simulink library "pixhawk_slib_swarm"  (R2022b)
settings: Solver=ode45  StartTime=0.0  StopTime=10.0  RelTol=1e-3
libraries: $bdroot x3, etargetslib x2, simulink x2
(part 2 of 2)

== system pixhawk_slib_swarm/RealCtrl28D/getMask6 ==
  In1 : Inport
  In2 : Inport  Port=2
  Data Type Conversion6 : DataTypeConversion  OutDataTypeStr=uint32  SaturateOnIntegerOverflow=off  RndMeth=Floor
  IgnoreAll : Constant  Value=bin2dec('1111111111111111')
  Switch : Switch  Criteria=u2 > Threshold  SaturateOnIntegerOverflow=off  InputSameDT=off
  Out1 : Outport  VectorParamsAs1DForOutWhenUnconnected=off
  wires:
  In1/1 -> Switch/2
  Switch/1 -> Data Type Conversion6/1
  Data Type Conversion6/1 -> Out1/1
  IgnoreAll/1 -> Switch/3
  In2/1 -> Switch/1

== system pixhawk_slib_swarm/RealCtrl28D/getMask7 ==
  In1 : Inport
  In2 : Inport  Port=2
  Data Type Conversion6 : DataTypeConversion  OutDataTypeStr=uint32  SaturateOnIntegerOverflow=off  RndMeth=Floor
  IgnoreAll : Constant  Value=bin2dec('1111111111111111')
  Switch : Switch  Criteria=u2 > Threshold  SaturateOnIntegerOverflow=off  InputSameDT=off
  Out1 : Outport  VectorParamsAs1DForOutWhenUnconnected=off
  wires:
  In1/1 -> Switch/2
  Switch/1 -> Data Type Conversion6/1
  Data Type Conversion6/1 -> Out1/1
  IgnoreAll/1 -> Switch/3
  In2/1 -> Switch/1

== system pixhawk_slib_swarm/RealCtrl28D/getMask8 ==
  In1 : Inport
  In2 : Inport  Port=2
  Data Type Conversion6 : DataTypeConversion  OutDataTypeStr=uint32  SaturateOnIntegerOverflow=off  RndMeth=Floor
  IgnoreAll : Constant  Value=bin2dec('1111111111111111')
  Switch : Switch  Criteria=u2 > Threshold  SaturateOnIntegerOverflow=off  InputSameDT=off
  Out1 : Outport  VectorParamsAs1DForOutWhenUnconnected=off
  wires:
  In1/1 -> Switch/2
  Switch/1 -> Data Type Conversion6/1
  Data Type Conversion6/1 -> Out1/1
  IgnoreAll/1 -> Switch/3
  In2/1 -> Switch/1

== system pixhawk_slib_swarm/RealCtrl28D/getMask9 ==
  In1 : Inport
  In2 : Inport  Port=2
  Data Type Conversion6 : DataTypeConversion  OutDataTypeStr=uint32  SaturateOnIntegerOverflow=off  RndMeth=Floor
  IgnoreAll : Constant  Value=bin2dec('1111111111111111')
  Switch : Switch  Criteria=u2 > Threshold  SaturateOnIntegerOverflow=off  InputSameDT=off
  Out1 : Outport  VectorParamsAs1DForOutWhenUnconnected=off
  wires:
  In1/1 -> Switch/2
  Switch/1 -> Data Type Conversion6/1
  Data Type Conversion6/1 -> Out1/1
  IgnoreAll/1 -> Switch/3
  In2/1 -> Switch/1

== matlab function pixhawk_slib_swarm/HighLevelMode/MATLAB Function ==
  data: ctrlCmd output; cmd input; mode input; ctrls input; takeoff_height input; status input; enableControl output; x output; y output; z output; vx output; clock input; vy output; vz output; accx output; accy output; accz output; yaw output; yawrate output
function [ctrlCmd, enableControl,x,y,z,vx,vy,vz,accx,accy,accz,yaw,yawrate] = fcn(cmd, mode, ctrls,takeoff_height, status, clock)
persistent last_send_t;
persistent send_interval;

if isempty(last_send_t)
    last_send_t = 0;
    % command will send with send_interval s.
    send_interval = 1;
end

ctrlCmd = cmd;
if cmd >0 && (clock-last_send_t>send_interval)
    last_send_t = clock;
    % The first bit determine whether has command, 1-has command, 0-ignore
    ctrlCmd = cmd + 1;
end

x = 0;
y = 0;
z = 0;
vx = 0;
vy = 0;
vz = 0;
accx = 0;
accy = 0;
accz = 0;
yaw = 0;
yawrate = 0;

if cmd == 512
    if mode == 1
        x = ctrls(1);
        y = ctrls(2);
        z = ctrls(3);
        yaw = ctrls(4);
    elseif mode == 2
        vx = ctrls(1);
        vy = ctrls(2);
        vz = ctrls(3);
        yawrate = ctrls(4);
    elseif mode == 3
        accx = ctrls(1);
        accy = ctrls(2);
        accz = ctrls(3);
        yawrate = ctrls(4);
    else
        disp("Not supported mode");
    end
end

if (cmd == 256) || (cmd == 512) || (cmd == 1024)|| (cmd == 128)
    enableControl = true;
else
    enableControl = false;
end

if cmd == 256
    % -0.2 is the minimum takeoff height
    if takeoff_height < -0.2
        z = takeoff_height; 
    end
end

if cmd == 1024
    z = 0;
end

if cmd == 128
    z = 0;
end

if ~ status
    ctrlCmd = uint32(0);
    enableControl = false;
    x = 0;
    y = 0;
    z = 0;
    vx = 0;
    vy = 0;
    vz = 0;
    accx = 0;
    accy = 0;
    accz = 0;
    yaw = 0;
    yawrate = 0;
end

== matlab function pixhawk_slib_swarm/Offboard_full/MATLAB Function ==
  data: pos input; y output; vel input; Acc input; Force input; Yaw input; Yawrate input
function y = fcn(pos,vel,Acc,Force,Yaw,Yawrate)
y=uint32(0);
if ~pos
    y = bitor(y,uint32(7));
end

if~vel
    y = bitor(y,bitshift(uint32(7),3));
end

if ~Acc
    y = bitor(y,bitshift(uint32(7),6));
end

if Force
    y = bitor(y,bitshift(uint32(1),9));
end

if ~Yaw
    y = bitor(y,bitshift(uint32(1),10));
end

if ~Yawrate
    y = bitor(y,bitshift(uint32(1),11));
end

== matlab function pixhawk_slib_swarm/real_data_decoder/Decoder1 ==
  data: u input; globalPos output; AngEular output; localPos output; localVel output; keyPressed output; selfCheckState output; isHeartRec output; TargetSysID output; TargetCompID output; isLocalNed output; isArmed output; isOffboard output; isFailSafeEn output; base_mode output; custom_mode output; system_status output; batteryInfo output; flyMode output; isStanby output; isActive output; isLowBatt output; isHighLoad output; isDropComm output; isGlobPos output; isGpsHome output; isSimorExe output; obstacle output
function [globalPos,AngEular,localPos,localVel,keyPressed,selfCheckState,isHeartRec,TargetSysID,TargetCompID,isLocalNed,isArmed,isOffboard,isFailSafeEn,base_mode,custom_mode,system_status,batteryInfo,flyMode,isStanby,isActive,isLowBatt,isHighLoad,isDropComm,isGlobPos,isGpsHome,isSimorExe,obstacle] = fcn(u)

globalPos=u(1:3);  % CopterSim全局位置，单位m。根据飞机的GPS坐标解算得到，以Ue地图的坐标中心为原点，使用多机控制时，应该使用本接口。
AngEular=u(4:6); %Pixhawk估计得到的以gpsHome为原点的相对北东地位置向量，单位m，z轴向下为正
localPos=u(7:9); %北东地的运动速度向量，单位m/s
localVel=u(10:12); %Pixhawk估计得到的姿态欧拉角，单位弧度

keyPressed=u(13);
selfCheckState=u(14);
isHeartRec=u(15);
TargetSysID=u(16);
TargetCompID=u(17);
isLocalNed=u(18);
isArmed=u(19);
isOffboard=u(20);
isFailSafeEn=u(21);
base_mode=u(22);
custom_mode=u(23);
system_status=u(24);
batteryInfo=u(25:27); %3D

flyMode=u(28);
isStanby=u(29);
isActive=u(30);
isLowBatt=u(31);
isHighLoad=u(32);
isDropComm=u(33);
isGlobPos=u(34);
isGpsHome=u(35);
isSimorExe=u(36);

obstacle=u(37:40); %[37] id for obstacle, [38-40] x,y,z position for obstacle

== matlab function pixhawk_slib_swarm/Full_data_decoder/Decoder1 ==
  data: u input; globalPos output; AngEular output; localPos output; localVel output; GpsPos output; GpsVel output; gpsHome output; time_boot_ms output; copterID output; relative_alt output; hdg output; satellites_visible output; fix_type output; resrveInit output; pos_horiz_accuracy output; pos_vert_accuracy output; resrveFloat output
function [globalPos,AngEular,localPos,localVel,GpsPos,GpsVel,gpsHome,time_boot_ms,copterID,relative_alt,hdg,satellites_visible,fix_type,resrveInit,pos_horiz_accuracy,pos_vert_accuracy,resrveFloat] = fcn(u)

globalPos=u(29:31);  % CopterSim全局位置，单位m。根据飞机的GPS坐标解算得到，以Ue地图的坐标中心为原点，使用多机控制时，应该使用本接口。
gpsHome=u(1:3);  %Home点（上电之后不会变）的经纬高坐标，经纬度需要除以1e7才能得到度为单位的经纬度，高需要除以1e3才能得到m为单位的高（向上为正）
AngEular=u(4:6); %Pixhawk估计得到的姿态欧拉角，单位弧度
localPos=u(7:9); %Pixhawk估计得到的以gpsHome为原点的相对北东地位置向量，单位m，z轴向下为正
localVel=u(10:12); %北东地的运动速度向量，单位m/s
GpsPos=u(13:15); %实时的GPS位置，单位和gpsHome相同，但是会实时变化
GpsVel=u(16:18); %GPS速度，需要除以100得到m/s为单位的速度
time_boot_ms=u(19);%上电时间
copterID=u(20);      %飞机ID
relative_alt=u(21); % GPS相对高度，需要除以1000得到m为单位的高度，向上为正
hdg=u(22); % GPS航向角，需要除以1000得到0~360度范围的角度
satellites_visible=u(23); %可见卫星数量
fix_type=u(24); %定位精度
resrveInit=u(25); % int类型的保留位
pos_horiz_accuracy=u(26); %水平定位精度，单位m
pos_vert_accuracy=u(27); %竖直定位精度，单位m
resrveFloat=u(28); % float型保留位，未被启用

== matlab function pixhawk_slib_swarm/vrpn_data_decoder/Decoder ==
  data: u input; t_pos output; pos_xyz output; quat_wxyz output; euler output; t_vel output; vel_xyz output; t_acc output; acc_xyz output; has_data output; has_pos output
function [t_pos,pos_xyz,quat_wxyz,euler,t_vel,vel_xyz,t_acc,acc_xyz,has_data,has_pos] = fcn(u)
% y0 -> Time stamp sec for pos msg
% y1 -> Time stamp usec for pos msg
% t_pos_msg = y0 + y1 / 1000000.0
% y2-y4 -> Pos_x,Pos_y,Pos_z in ned, unit m
% y5-y8 -> Quat (w,x,y,z) for vehicle attitude
% y9 -> Time stamp sec for vel msg
% y10 -> Time stamp usec for vel msg
% t_vel_msg = y9 + y10 / 1000000.0
% y11-y13 -> vel_x,vel_y,vel_z in ned, unit m/s
% y14 -> Time stamp sec for acc msg
% y15 -> Time stamp usec for acc msg
% y16-y18 -> acc_x,acc_y,acc_z in ned, unit m/s^2
% y19-y21 -> Euler (roll pitch yaw) ang from vehicle Quat
% y22 -> tracker->has_data, is there any vrpn message received.
% y23 -> tracker->has_pos, is the vrpn pos message received.
% 24-29 -> reserve for future use

t_pos=u(1)+u(2)/1000000.0;
pos_xyz=u(3:5);
quat_wxyz=u(6:9);
t_vel=u(10)+u(11)/1000000.0;
vel_xyz=u(12:14);
t_acc=u(15)+u(16)/1000000.0;
acc_xyz=u(17:19);
euler=u(20:22);
has_data = u(23);
has_pos = u(24);
